simulink model "chap10_6"  (Simulink 3.00)
settings: Solver=ode45  StartTime=0.0  StopTime=20  FixedStep=0.001  RelTol=1e-3

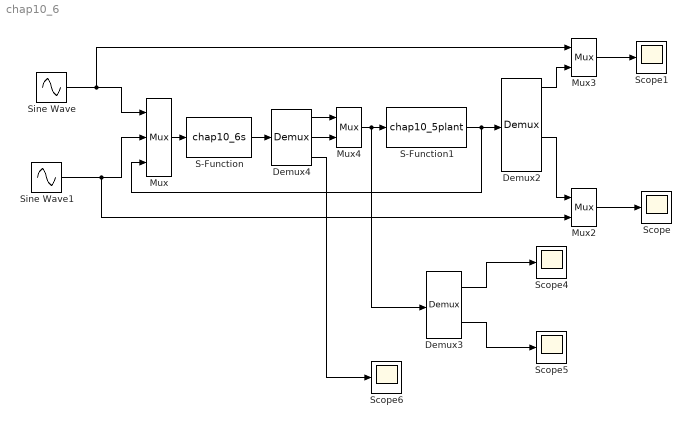
== system chap10_6 ==
  Demux2 : Demux  Outputs=4
  Demux3 : Demux  Outputs=2
  Demux4 : Demux  Outputs=3
  Mux : Mux  Inputs=3
      settings: DisplayOption=none
  Mux2 : Mux  Inputs=2
      settings: DisplayOption=none
  Mux3 : Mux  Inputs=2
      settings: DisplayOption=none
  Mux4 : Mux  Inputs=2
      settings: DisplayOption=none
  S-Function : S-Function  FunctionName=chap10_6s  PortCounts=[]  SFunctionModules=''
  S-Function1 : S-Function  FunctionName=chap10_5plant  PortCounts=[]  SFunctionModules=''
  Scope{,1,4..6} (5 alike) : Scope
      Scope settings: TickLabels=on  TimeRange=4  YMin=0  YMax=37500  SaveToWorkspace=off  SaveName=ScopeData  MaxRows=50000
      Scope1 settings: TimeRange=auto  YMin=-1.1  YMax=1  SaveToWorkspace=off  SaveName=ScopeData  MaxRows=50000
      Scope4 settings: TickLabels=on  TimeRange=4  YMin=-350  YMax=600  SaveToWorkspace=off  SaveName=ScopeData  MaxRows=50000
      Scope5 settings: TickLabels=on  TimeRange=4  YMin=-1  YMax=1  SaveToWorkspace=off  SaveName=ScopeData  MaxRows=50000
      Scope6 settings: TickLabels=on  TimeRange=4  YMin=-7.5  YMax=-2.75  SaveToWorkspace=off  SaveName=ScopeData  MaxRows=50000
  Sine Wave : Sin  Amplitude=1  Frequency=pi  Phase=pi/2  SampleTime=0
  Sine Wave1 : Sin  Amplitude=1  Frequency=pi  Phase=0  SampleTime=0
  wires:
  Mux/1 -> S-Function/1
  Mux3/1 -> Scope1/1
  S-Function/1 -> Demux4/1
  Demux4/1 -> Mux4/1
  Demux4/2 -> Mux4/2
  Mux2/1 -> Scope/1
  Demux4/3 -> Scope6/1
  Demux3/1 -> Scope4/1
  Demux3/2 -> Scope5/1
  Demux2/3 -> Mux2/1
  Demux2/1 -> Mux3/2
  S-Function1/1 -> Demux2/1, Mux/3
  Mux4/1 -> S-Function1/1, Demux3/1
  Sine Wave/1 -> Mux/1, Mux3/1
  Sine Wave1/1 -> Mux/2, Mux2/2
